simulink library "lib_decmp_Calib_tbm_ctr_x8"  (R2020a)
settings: Solver=VariableStepAuto  StartTime=0.0  StopTime=10.0  RelTol=1e-3
settings Model: Creator=Administrator  LastModifiedBy=Administrator

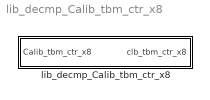
== system lib_decmp_Calib_tbm_ctr_x8 ==
  lib_decmp_Calib_tbm_ctr_x8 : Subsystem

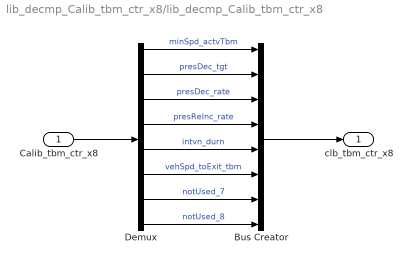
== system lib_decmp_Calib_tbm_ctr_x8/lib_decmp_Calib_tbm_ctr_x8 ==
  Calib_tbm_ctr_x8 : Inport  OutDataTypeStr=single  PortDimensions=8
  Bus Creator : BusCreator  Inputs=8
  Demux : Demux  Outputs=8
  clb_tbm_ctr_x8 : Outport  PortDimensions=8
  wires:
  Calib_tbm_ctr_x8/1 -> Demux/1
  Demux/1 -> Bus Creator/1  "minSpd_actvTbm"
  Demux/2 -> Bus Creator/2  "presDec_tgt"
  Demux/3 -> Bus Creator/3  "presDec_rate"
  Demux/4 -> Bus Creator/4  "presReInc_rate"
  Bus Creator/1 -> clb_tbm_ctr_x8/1
  Demux/5 -> Bus Creator/5  "intvn_durn"
  Demux/6 -> Bus Creator/6  "vehSpd_toExit_tbm"
  Demux/7 -> Bus Creator/7  "notUsed_7"
  Demux/8 -> Bus Creator/8  "notUsed_8"
